simulink model "PROGRAM_COUNTER_02"  (R2022a)
settings: Solver=VariableStepAuto  StartTime=0.0  StopTime=10.0  RelTol=1e-3
undefined symbols (not defined in the file or in its folder): xc7z010iclg225
libraries: hdlBasic x1933, hlsBasic x1, vmcUtilities x1
(part 9 of 12)

== system PROGRAM_COUNTER_02/SUMADOR_64_BITS_1/ALU_SUM_18 ==
  CARRY_IN (1 BIT) : Inport
  A_INPUT (1 BIT) : Inport  Port=2
  B_INPUT (1 BIT) : Inport  Port=3
  Inverter1 : hdlBasic/Inverter  en=off  latency=0  XmcBlockStatus=1  maskContainerNames=group2  block_type=inv  block_config=sysgen:Inverter_config
  Inverter8 : hdlBasic/Inverter  en=off  latency=0  XmcBlockStatus=1  maskContainerNames=group2  block_type=inv  block_config=sysgen:Inverter_config
  Inverter9 : hdlBasic/Inverter  en=off  latency=0  XmcBlockStatus=1  maskContainerNames=group2  block_type=inv  block_config=sysgen:Inverter_config
  Logical : hdlBasic/Logical  logical_function=AND  inputs=2  en=off  latency=0  precision=Full  arith_type=Unsigned  n_bits=16  bin_pt=0  align_bp=on  overflow=[]  quantization=[]  XmcBlockStatus=1  maskContainerNames=tabcontainer1  block_type=logical  block_config=sysgen:Logical_config
  Logical1 : hdlBasic/Logical  logical_function=AND  inputs=2  en=off  latency=0  precision=Full  arith_type=Unsigned  n_bits=16  bin_pt=0  align_bp=on  overflow=[]  quantization=[]  XmcBlockStatus=1  maskContainerNames=tabcontainer1  block_type=logical  block_config=sysgen:Logical_config
  Logical2 : hdlBasic/Logical  logical_function=AND  inputs=2  en=off  latency=0  precision=Full  arith_type=Unsigned  n_bits=16  bin_pt=0  align_bp=on  overflow=[]  quantization=[]  XmcBlockStatus=1  maskContainerNames=tabcontainer1  block_type=logical  block_config=sysgen:Logical_config
  Logical{4..6,9} (4 alike) : hdlBasic/Logical  logical_function=AND  inputs=3  en=off  latency=0  precision=Full  arith_type=Unsigned  n_bits=16  bin_pt=0  align_bp=on  overflow=[]  quantization=[]  XmcBlockStatus=1  maskContainerNames=tabcontainer1  block_type=logical  block_config=sysgen:Logical_config
  Sum : hdlBasic/Logical  logical_function=OR  inputs=4  en=off  latency=0  precision=Full  arith_type=Unsigned  n_bits=16  bin_pt=0  align_bp=on  overflow=[]  quantization=[]  XmcBlockStatus=1  maskContainerNames=tabcontainer1  block_type=logical  block_config=sysgen:Logical_config
  c_out : hdlBasic/Logical  logical_function=OR  inputs=3  en=off  latency=0  precision=Full  arith_type=Unsigned  n_bits=16  bin_pt=0  align_bp=on  overflow=[]  quantization=[]  XmcBlockStatus=1  maskContainerNames=tabcontainer1  block_type=logical  block_config=sysgen:Logical_config
  ALU_OUT (1 BIT) : Outport
  CARRY_OUT (1 BIT) : Outport  Port=2
  wires:
  A_INPUT (1 BIT)/1 -> Inverter8/1, Logical5/2, Logical/2, Logical2/1, Logical9/2
  Logical1/1 -> c_out/2
  Inverter8/1 -> Logical6/2, Logical4/2
  CARRY_IN (1 BIT)/1 -> Inverter1/1, Logical5/1, Logical4/1, Logical1/1, Logical/1
  B_INPUT (1 BIT)/1 -> Logical5/3, Logical6/3, Logical1/2, Logical2/2, Inverter9/1
  Inverter1/1 -> Logical6/1, Logical9/1
  Logical6/1 -> Sum/3
  Logical9/1 -> Sum/2
  Logical4/1 -> Sum/1
  Logical/1 -> c_out/1
  Logical5/1 -> Sum/4
  Inverter9/1 -> Logical9/3, Logical4/3
  Sum/1 -> ALU_OUT (1 BIT)/1
  Logical2/1 -> c_out/3
  c_out/1 -> CARRY_OUT (1 BIT)/1

== system PROGRAM_COUNTER_02/SUMADOR_64_BITS_1/ALU_SUM_19 ==
  CARRY_IN (1 BIT) : Inport
  A_INPUT (1 BIT) : Inport  Port=2
  B_INPUT (1 BIT) : Inport  Port=3
  Inverter1 : hdlBasic/Inverter  en=off  latency=0  XmcBlockStatus=1  maskContainerNames=group2  block_type=inv  block_config=sysgen:Inverter_config
  Inverter8 : hdlBasic/Inverter  en=off  latency=0  XmcBlockStatus=1  maskContainerNames=group2  block_type=inv  block_config=sysgen:Inverter_config
  Inverter9 : hdlBasic/Inverter  en=off  latency=0  XmcBlockStatus=1  maskContainerNames=group2  block_type=inv  block_config=sysgen:Inverter_config
  Logical : hdlBasic/Logical  logical_function=AND  inputs=2  en=off  latency=0  precision=Full  arith_type=Unsigned  n_bits=16  bin_pt=0  align_bp=on  overflow=[]  quantization=[]  XmcBlockStatus=1  maskContainerNames=tabcontainer1  block_type=logical  block_config=sysgen:Logical_config
  Logical1 : hdlBasic/Logical  logical_function=AND  inputs=2  en=off  latency=0  precision=Full  arith_type=Unsigned  n_bits=16  bin_pt=0  align_bp=on  overflow=[]  quantization=[]  XmcBlockStatus=1  maskContainerNames=tabcontainer1  block_type=logical  block_config=sysgen:Logical_config
  Logical2 : hdlBasic/Logical  logical_function=AND  inputs=2  en=off  latency=0  precision=Full  arith_type=Unsigned  n_bits=16  bin_pt=0  align_bp=on  overflow=[]  quantization=[]  XmcBlockStatus=1  maskContainerNames=tabcontainer1  block_type=logical  block_config=sysgen:Logical_config
  Logical{4..6,9} (4 alike) : hdlBasic/Logical  logical_function=AND  inputs=3  en=off  latency=0  precision=Full  arith_type=Unsigned  n_bits=16  bin_pt=0  align_bp=on  overflow=[]  quantization=[]  XmcBlockStatus=1  maskContainerNames=tabcontainer1  block_type=logical  block_config=sysgen:Logical_config
  Sum : hdlBasic/Logical  logical_function=OR  inputs=4  en=off  latency=0  precision=Full  arith_type=Unsigned  n_bits=16  bin_pt=0  align_bp=on  overflow=[]  quantization=[]  XmcBlockStatus=1  maskContainerNames=tabcontainer1  block_type=logical  block_config=sysgen:Logical_config
  c_out : hdlBasic/Logical  logical_function=OR  inputs=3  en=off  latency=0  precision=Full  arith_type=Unsigned  n_bits=16  bin_pt=0  align_bp=on  overflow=[]  quantization=[]  XmcBlockStatus=1  maskContainerNames=tabcontainer1  block_type=logical  block_config=sysgen:Logical_config
  ALU_OUT (1 BIT) : Outport
  CARRY_OUT (1 BIT) : Outport  Port=2
  wires:
  A_INPUT (1 BIT)/1 -> Inverter8/1, Logical5/2, Logical/2, Logical2/1, Logical9/2
  Logical1/1 -> c_out/2
  Inverter8/1 -> Logical6/2, Logical4/2
  CARRY_IN (1 BIT)/1 -> Inverter1/1, Logical5/1, Logical4/1, Logical1/1, Logical/1
  B_INPUT (1 BIT)/1 -> Logical5/3, Logical6/3, Logical1/2, Logical2/2, Inverter9/1
  Inverter1/1 -> Logical6/1, Logical9/1
  Logical6/1 -> Sum/3
  Logical9/1 -> Sum/2
  Logical4/1 -> Sum/1
  Logical/1 -> c_out/1
  Logical5/1 -> Sum/4
  Inverter9/1 -> Logical9/3, Logical4/3
  Sum/1 -> ALU_OUT (1 BIT)/1
  Logical2/1 -> c_out/3
  c_out/1 -> CARRY_OUT (1 BIT)/1

== system PROGRAM_COUNTER_02/SUMADOR_64_BITS_1/ALU_SUM_2 ==
  CARRY_IN (1 BIT) : Inport
  A_INPUT (1 BIT) : Inport  Port=2
  B_INPUT (1 BIT) : Inport  Port=3
  Inverter1 : hdlBasic/Inverter  en=off  latency=0  XmcBlockStatus=1  maskContainerNames=group2  block_type=inv  block_config=sysgen:Inverter_config
  Inverter8 : hdlBasic/Inverter  en=off  latency=0  XmcBlockStatus=1  maskContainerNames=group2  block_type=inv  block_config=sysgen:Inverter_config
  Inverter9 : hdlBasic/Inverter  en=off  latency=0  XmcBlockStatus=1  maskContainerNames=group2  block_type=inv  block_config=sysgen:Inverter_config
  Logical : hdlBasic/Logical  logical_function=AND  inputs=2  en=off  latency=0  precision=Full  arith_type=Unsigned  n_bits=16  bin_pt=0  align_bp=on  overflow=[]  quantization=[]  XmcBlockStatus=1  maskContainerNames=tabcontainer1  block_type=logical  block_config=sysgen:Logical_config
  Logical1 : hdlBasic/Logical  logical_function=AND  inputs=2  en=off  latency=0  precision=Full  arith_type=Unsigned  n_bits=16  bin_pt=0  align_bp=on  overflow=[]  quantization=[]  XmcBlockStatus=1  maskContainerNames=tabcontainer1  block_type=logical  block_config=sysgen:Logical_config
  Logical2 : hdlBasic/Logical  logical_function=AND  inputs=2  en=off  latency=0  precision=Full  arith_type=Unsigned  n_bits=16  bin_pt=0  align_bp=on  overflow=[]  quantization=[]  XmcBlockStatus=1  maskContainerNames=tabcontainer1  block_type=logical  block_config=sysgen:Logical_config
  Logical{4..6,9} (4 alike) : hdlBasic/Logical  logical_function=AND  inputs=3  en=off  latency=0  precision=Full  arith_type=Unsigned  n_bits=16  bin_pt=0  align_bp=on  overflow=[]  quantization=[]  XmcBlockStatus=1  maskContainerNames=tabcontainer1  block_type=logical  block_config=sysgen:Logical_config
  Sum : hdlBasic/Logical  logical_function=OR  inputs=4  en=off  latency=0  precision=Full  arith_type=Unsigned  n_bits=16  bin_pt=0  align_bp=on  overflow=[]  quantization=[]  XmcBlockStatus=1  maskContainerNames=tabcontainer1  block_type=logical  block_config=sysgen:Logical_config
  c_out : hdlBasic/Logical  logical_function=OR  inputs=3  en=off  latency=0  precision=Full  arith_type=Unsigned  n_bits=16  bin_pt=0  align_bp=on  overflow=[]  quantization=[]  XmcBlockStatus=1  maskContainerNames=tabcontainer1  block_type=logical  block_config=sysgen:Logical_config
  ALU_OUT (1 BIT) : Outport
  CARRY_OUT (1 BIT) : Outport  Port=2
  wires:
  A_INPUT (1 BIT)/1 -> Inverter8/1, Logical5/2, Logical/2, Logical2/1, Logical9/2
  Logical1/1 -> c_out/2
  Inverter8/1 -> Logical6/2, Logical4/2
  CARRY_IN (1 BIT)/1 -> Inverter1/1, Logical5/1, Logical4/1, Logical1/1, Logical/1
  B_INPUT (1 BIT)/1 -> Logical5/3, Logical6/3, Logical1/2, Logical2/2, Inverter9/1
  Inverter1/1 -> Logical6/1, Logical9/1
  Logical6/1 -> Sum/3
  Logical9/1 -> Sum/2
  Logical4/1 -> Sum/1
  Logical/1 -> c_out/1
  Logical5/1 -> Sum/4
  Inverter9/1 -> Logical9/3, Logical4/3
  Sum/1 -> ALU_OUT (1 BIT)/1
  Logical2/1 -> c_out/3
  c_out/1 -> CARRY_OUT (1 BIT)/1

== system PROGRAM_COUNTER_02/SUMADOR_64_BITS_1/ALU_SUM_20 ==
  CARRY_IN (1 BIT) : Inport
  A_INPUT (1 BIT) : Inport  Port=2
  B_INPUT (1 BIT) : Inport  Port=3
  Inverter1 : hdlBasic/Inverter  en=off  latency=0  XmcBlockStatus=1  maskContainerNames=group2  block_type=inv  block_config=sysgen:Inverter_config
  Inverter8 : hdlBasic/Inverter  en=off  latency=0  XmcBlockStatus=1  maskContainerNames=group2  block_type=inv  block_config=sysgen:Inverter_config
  Inverter9 : hdlBasic/Inverter  en=off  latency=0  XmcBlockStatus=1  maskContainerNames=group2  block_type=inv  block_config=sysgen:Inverter_config
  Logical : hdlBasic/Logical  logical_function=AND  inputs=2  en=off  latency=0  precision=Full  arith_type=Unsigned  n_bits=16  bin_pt=0  align_bp=on  overflow=[]  quantization=[]  XmcBlockStatus=1  maskContainerNames=tabcontainer1  block_type=logical  block_config=sysgen:Logical_config
  Logical1 : hdlBasic/Logical  logical_function=AND  inputs=2  en=off  latency=0  precision=Full  arith_type=Unsigned  n_bits=16  bin_pt=0  align_bp=on  overflow=[]  quantization=[]  XmcBlockStatus=1  maskContainerNames=tabcontainer1  block_type=logical  block_config=sysgen:Logical_config
  Logical2 : hdlBasic/Logical  logical_function=AND  inputs=2  en=off  latency=0  precision=Full  arith_type=Unsigned  n_bits=16  bin_pt=0  align_bp=on  overflow=[]  quantization=[]  XmcBlockStatus=1  maskContainerNames=tabcontainer1  block_type=logical  block_config=sysgen:Logical_config
  Logical{4..6,9} (4 alike) : hdlBasic/Logical  logical_function=AND  inputs=3  en=off  latency=0  precision=Full  arith_type=Unsigned  n_bits=16  bin_pt=0  align_bp=on  overflow=[]  quantization=[]  XmcBlockStatus=1  maskContainerNames=tabcontainer1  block_type=logical  block_config=sysgen:Logical_config
  Sum : hdlBasic/Logical  logical_function=OR  inputs=4  en=off  latency=0  precision=Full  arith_type=Unsigned  n_bits=16  bin_pt=0  align_bp=on  overflow=[]  quantization=[]  XmcBlockStatus=1  maskContainerNames=tabcontainer1  block_type=logical  block_config=sysgen:Logical_config
  c_out : hdlBasic/Logical  logical_function=OR  inputs=3  en=off  latency=0  precision=Full  arith_type=Unsigned  n_bits=16  bin_pt=0  align_bp=on  overflow=[]  quantization=[]  XmcBlockStatus=1  maskContainerNames=tabcontainer1  block_type=logical  block_config=sysgen:Logical_config
  ALU_OUT (1 BIT) : Outport
  CARRY_OUT (1 BIT) : Outport  Port=2
  wires:
  A_INPUT (1 BIT)/1 -> Inverter8/1, Logical5/2, Logical/2, Logical2/1, Logical9/2
  Logical1/1 -> c_out/2
  Inverter8/1 -> Logical6/2, Logical4/2
  CARRY_IN (1 BIT)/1 -> Inverter1/1, Logical5/1, Logical4/1, Logical1/1, Logical/1
  B_INPUT (1 BIT)/1 -> Logical5/3, Logical6/3, Logical1/2, Logical2/2, Inverter9/1
  Inverter1/1 -> Logical6/1, Logical9/1
  Logical6/1 -> Sum/3
  Logical9/1 -> Sum/2
  Logical4/1 -> Sum/1
  Logical/1 -> c_out/1
  Logical5/1 -> Sum/4
  Inverter9/1 -> Logical9/3, Logical4/3
  Sum/1 -> ALU_OUT (1 BIT)/1
  Logical2/1 -> c_out/3
  c_out/1 -> CARRY_OUT (1 BIT)/1

== system PROGRAM_COUNTER_02/SUMADOR_64_BITS_1/ALU_SUM_21 ==
  CARRY_IN (1 BIT) : Inport
  A_INPUT (1 BIT) : Inport  Port=2
  B_INPUT (1 BIT) : Inport  Port=3
  Inverter1 : hdlBasic/Inverter  en=off  latency=0  XmcBlockStatus=1  maskContainerNames=group2  block_type=inv  block_config=sysgen:Inverter_config
  Inverter8 : hdlBasic/Inverter  en=off  latency=0  XmcBlockStatus=1  maskContainerNames=group2  block_type=inv  block_config=sysgen:Inverter_config
  Inverter9 : hdlBasic/Inverter  en=off  latency=0  XmcBlockStatus=1  maskContainerNames=group2  block_type=inv  block_config=sysgen:Inverter_config
  Logical : hdlBasic/Logical  logical_function=AND  inputs=2  en=off  latency=0  precision=Full  arith_type=Unsigned  n_bits=16  bin_pt=0  align_bp=on  overflow=[]  quantization=[]  XmcBlockStatus=1  maskContainerNames=tabcontainer1  block_type=logical  block_config=sysgen:Logical_config
  Logical1 : hdlBasic/Logical  logical_function=AND  inputs=2  en=off  latency=0  precision=Full  arith_type=Unsigned  n_bits=16  bin_pt=0  align_bp=on  overflow=[]  quantization=[]  XmcBlockStatus=1  maskContainerNames=tabcontainer1  block_type=logical  block_config=sysgen:Logical_config
  Logical2 : hdlBasic/Logical  logical_function=AND  inputs=2  en=off  latency=0  precision=Full  arith_type=Unsigned  n_bits=16  bin_pt=0  align_bp=on  overflow=[]  quantization=[]  XmcBlockStatus=1  maskContainerNames=tabcontainer1  block_type=logical  block_config=sysgen:Logical_config
  Logical{4..6,9} (4 alike) : hdlBasic/Logical  logical_function=AND  inputs=3  en=off  latency=0  precision=Full  arith_type=Unsigned  n_bits=16  bin_pt=0  align_bp=on  overflow=[]  quantization=[]  XmcBlockStatus=1  maskContainerNames=tabcontainer1  block_type=logical  block_config=sysgen:Logical_config
  Sum : hdlBasic/Logical  logical_function=OR  inputs=4  en=off  latency=0  precision=Full  arith_type=Unsigned  n_bits=16  bin_pt=0  align_bp=on  overflow=[]  quantization=[]  XmcBlockStatus=1  maskContainerNames=tabcontainer1  block_type=logical  block_config=sysgen:Logical_config
  c_out : hdlBasic/Logical  logical_function=OR  inputs=3  en=off  latency=0  precision=Full  arith_type=Unsigned  n_bits=16  bin_pt=0  align_bp=on  overflow=[]  quantization=[]  XmcBlockStatus=1  maskContainerNames=tabcontainer1  block_type=logical  block_config=sysgen:Logical_config
  ALU_OUT (1 BIT) : Outport
  CARRY_OUT (1 BIT) : Outport  Port=2
  wires:
  A_INPUT (1 BIT)/1 -> Inverter8/1, Logical5/2, Logical/2, Logical2/1, Logical9/2
  Logical1/1 -> c_out/2
  Inverter8/1 -> Logical6/2, Logical4/2
  CARRY_IN (1 BIT)/1 -> Inverter1/1, Logical5/1, Logical4/1, Logical1/1, Logical/1
  B_INPUT (1 BIT)/1 -> Logical5/3, Logical6/3, Logical1/2, Logical2/2, Inverter9/1
  Inverter1/1 -> Logical6/1, Logical9/1
  Logical6/1 -> Sum/3
  Logical9/1 -> Sum/2
  Logical4/1 -> Sum/1
  Logical/1 -> c_out/1
  Logical5/1 -> Sum/4
  Inverter9/1 -> Logical9/3, Logical4/3
  Sum/1 -> ALU_OUT (1 BIT)/1
  Logical2/1 -> c_out/3
  c_out/1 -> CARRY_OUT (1 BIT)/1

== system PROGRAM_COUNTER_02/SUMADOR_64_BITS_1/ALU_SUM_22 ==
  CARRY_IN (1 BIT) : Inport
  A_INPUT (1 BIT) : Inport  Port=2
  B_INPUT (1 BIT) : Inport  Port=3
  Inverter1 : hdlBasic/Inverter  en=off  latency=0  XmcBlockStatus=1  maskContainerNames=group2  block_type=inv  block_config=sysgen:Inverter_config
  Inverter8 : hdlBasic/Inverter  en=off  latency=0  XmcBlockStatus=1  maskContainerNames=group2  block_type=inv  block_config=sysgen:Inverter_config
  Inverter9 : hdlBasic/Inverter  en=off  latency=0  XmcBlockStatus=1  maskContainerNames=group2  block_type=inv  block_config=sysgen:Inverter_config
  Logical : hdlBasic/Logical  logical_function=AND  inputs=2  en=off  latency=0  precision=Full  arith_type=Unsigned  n_bits=16  bin_pt=0  align_bp=on  overflow=[]  quantization=[]  XmcBlockStatus=1  maskContainerNames=tabcontainer1  block_type=logical  block_config=sysgen:Logical_config
  Logical1 : hdlBasic/Logical  logical_function=AND  inputs=2  en=off  latency=0  precision=Full  arith_type=Unsigned  n_bits=16  bin_pt=0  align_bp=on  overflow=[]  quantization=[]  XmcBlockStatus=1  maskContainerNames=tabcontainer1  block_type=logical  block_config=sysgen:Logical_config
  Logical2 : hdlBasic/Logical  logical_function=AND  inputs=2  en=off  latency=0  precision=Full  arith_type=Unsigned  n_bits=16  bin_pt=0  align_bp=on  overflow=[]  quantization=[]  XmcBlockStatus=1  maskContainerNames=tabcontainer1  block_type=logical  block_config=sysgen:Logical_config
  Logical{4..6,9} (4 alike) : hdlBasic/Logical  logical_function=AND  inputs=3  en=off  latency=0  precision=Full  arith_type=Unsigned  n_bits=16  bin_pt=0  align_bp=on  overflow=[]  quantization=[]  XmcBlockStatus=1  maskContainerNames=tabcontainer1  block_type=logical  block_config=sysgen:Logical_config
  Sum : hdlBasic/Logical  logical_function=OR  inputs=4  en=off  latency=0  precision=Full  arith_type=Unsigned  n_bits=16  bin_pt=0  align_bp=on  overflow=[]  quantization=[]  XmcBlockStatus=1  maskContainerNames=tabcontainer1  block_type=logical  block_config=sysgen:Logical_config
  c_out : hdlBasic/Logical  logical_function=OR  inputs=3  en=off  latency=0  precision=Full  arith_type=Unsigned  n_bits=16  bin_pt=0  align_bp=on  overflow=[]  quantization=[]  XmcBlockStatus=1  maskContainerNames=tabcontainer1  block_type=logical  block_config=sysgen:Logical_config
  ALU_OUT (1 BIT) : Outport
  CARRY_OUT (1 BIT) : Outport  Port=2
  wires:
  A_INPUT (1 BIT)/1 -> Inverter8/1, Logical5/2, Logical/2, Logical2/1, Logical9/2
  Logical1/1 -> c_out/2
  Inverter8/1 -> Logical6/2, Logical4/2
  CARRY_IN (1 BIT)/1 -> Inverter1/1, Logical5/1, Logical4/1, Logical1/1, Logical/1
  B_INPUT (1 BIT)/1 -> Logical5/3, Logical6/3, Logical1/2, Logical2/2, Inverter9/1
  Inverter1/1 -> Logical6/1, Logical9/1
  Logical6/1 -> Sum/3
  Logical9/1 -> Sum/2
  Logical4/1 -> Sum/1
  Logical/1 -> c_out/1
  Logical5/1 -> Sum/4
  Inverter9/1 -> Logical9/3, Logical4/3
  Sum/1 -> ALU_OUT (1 BIT)/1
  Logical2/1 -> c_out/3
  c_out/1 -> CARRY_OUT (1 BIT)/1

== system PROGRAM_COUNTER_02/SUMADOR_64_BITS_1/ALU_SUM_23 ==
  CARRY_IN (1 BIT) : Inport
  A_INPUT (1 BIT) : Inport  Port=2
  B_INPUT (1 BIT) : Inport  Port=3
  Inverter1 : hdlBasic/Inverter  en=off  latency=0  XmcBlockStatus=1  maskContainerNames=group2  block_type=inv  block_config=sysgen:Inverter_config
  Inverter8 : hdlBasic/Inverter  en=off  latency=0  XmcBlockStatus=1  maskContainerNames=group2  block_type=inv  block_config=sysgen:Inverter_config
  Inverter9 : hdlBasic/Inverter  en=off  latency=0  XmcBlockStatus=1  maskContainerNames=group2  block_type=inv  block_config=sysgen:Inverter_config
  Logical : hdlBasic/Logical  logical_function=AND  inputs=2  en=off  latency=0  precision=Full  arith_type=Unsigned  n_bits=16  bin_pt=0  align_bp=on  overflow=[]  quantization=[]  XmcBlockStatus=1  maskContainerNames=tabcontainer1  block_type=logical  block_config=sysgen:Logical_config
  Logical1 : hdlBasic/Logical  logical_function=AND  inputs=2  en=off  latency=0  precision=Full  arith_type=Unsigned  n_bits=16  bin_pt=0  align_bp=on  overflow=[]  quantization=[]  XmcBlockStatus=1  maskContainerNames=tabcontainer1  block_type=logical  block_config=sysgen:Logical_config
  Logical2 : hdlBasic/Logical  logical_function=AND  inputs=2  en=off  latency=0  precision=Full  arith_type=Unsigned  n_bits=16  bin_pt=0  align_bp=on  overflow=[]  quantization=[]  XmcBlockStatus=1  maskContainerNames=tabcontainer1  block_type=logical  block_config=sysgen:Logical_config
  Logical{4..6,9} (4 alike) : hdlBasic/Logical  logical_function=AND  inputs=3  en=off  latency=0  precision=Full  arith_type=Unsigned  n_bits=16  bin_pt=0  align_bp=on  overflow=[]  quantization=[]  XmcBlockStatus=1  maskContainerNames=tabcontainer1  block_type=logical  block_config=sysgen:Logical_config
  Sum : hdlBasic/Logical  logical_function=OR  inputs=4  en=off  latency=0  precision=Full  arith_type=Unsigned  n_bits=16  bin_pt=0  align_bp=on  overflow=[]  quantization=[]  XmcBlockStatus=1  maskContainerNames=tabcontainer1  block_type=logical  block_config=sysgen:Logical_config
  c_out : hdlBasic/Logical  logical_function=OR  inputs=3  en=off  latency=0  precision=Full  arith_type=Unsigned  n_bits=16  bin_pt=0  align_bp=on  overflow=[]  quantization=[]  XmcBlockStatus=1  maskContainerNames=tabcontainer1  block_type=logical  block_config=sysgen:Logical_config
  ALU_OUT (1 BIT) : Outport
  CARRY_OUT (1 BIT) : Outport  Port=2
  wires:
  A_INPUT (1 BIT)/1 -> Inverter8/1, Logical5/2, Logical/2, Logical2/1, Logical9/2
  Logical1/1 -> c_out/2
  Inverter8/1 -> Logical6/2, Logical4/2
  CARRY_IN (1 BIT)/1 -> Inverter1/1, Logical5/1, Logical4/1, Logical1/1, Logical/1
  B_INPUT (1 BIT)/1 -> Logical5/3, Logical6/3, Logical1/2, Logical2/2, Inverter9/1
  Inverter1/1 -> Logical6/1, Logical9/1
  Logical6/1 -> Sum/3
  Logical9/1 -> Sum/2
  Logical4/1 -> Sum/1
  Logical/1 -> c_out/1
  Logical5/1 -> Sum/4
  Inverter9/1 -> Logical9/3, Logical4/3
  Sum/1 -> ALU_OUT (1 BIT)/1
  Logical2/1 -> c_out/3
  c_out/1 -> CARRY_OUT (1 BIT)/1

== system PROGRAM_COUNTER_02/SUMADOR_64_BITS_1/ALU_SUM_24 ==
  CARRY_IN (1 BIT) : Inport
  A_INPUT (1 BIT) : Inport  Port=2
  B_INPUT (1 BIT) : Inport  Port=3
  Inverter1 : hdlBasic/Inverter  en=off  latency=0  XmcBlockStatus=1  maskContainerNames=group2  block_type=inv  block_config=sysgen:Inverter_config
  Inverter8 : hdlBasic/Inverter  en=off  latency=0  XmcBlockStatus=1  maskContainerNames=group2  block_type=inv  block_config=sysgen:Inverter_config
  Inverter9 : hdlBasic/Inverter  en=off  latency=0  XmcBlockStatus=1  maskContainerNames=group2  block_type=inv  block_config=sysgen:Inverter_config
  Logical : hdlBasic/Logical  logical_function=AND  inputs=2  en=off  latency=0  precision=Full  arith_type=Unsigned  n_bits=16  bin_pt=0  align_bp=on  overflow=[]  quantization=[]  XmcBlockStatus=1  maskContainerNames=tabcontainer1  block_type=logical  block_config=sysgen:Logical_config
  Logical1 : hdlBasic/Logical  logical_function=AND  inputs=2  en=off  latency=0  precision=Full  arith_type=Unsigned  n_bits=16  bin_pt=0  align_bp=on  overflow=[]  quantization=[]  XmcBlockStatus=1  maskContainerNames=tabcontainer1  block_type=logical  block_config=sysgen:Logical_config
  Logical2 : hdlBasic/Logical  logical_function=AND  inputs=2  en=off  latency=0  precision=Full  arith_type=Unsigned  n_bits=16  bin_pt=0  align_bp=on  overflow=[]  quantization=[]  XmcBlockStatus=1  maskContainerNames=tabcontainer1  block_type=logical  block_config=sysgen:Logical_config
  Logical{4..6,9} (4 alike) : hdlBasic/Logical  logical_function=AND  inputs=3  en=off  latency=0  precision=Full  arith_type=Unsigned  n_bits=16  bin_pt=0  align_bp=on  overflow=[]  quantization=[]  XmcBlockStatus=1  maskContainerNames=tabcontainer1  block_type=logical  block_config=sysgen:Logical_config
  Sum : hdlBasic/Logical  logical_function=OR  inputs=4  en=off  latency=0  precision=Full  arith_type=Unsigned  n_bits=16  bin_pt=0  align_bp=on  overflow=[]  quantization=[]  XmcBlockStatus=1  maskContainerNames=tabcontainer1  block_type=logical  block_config=sysgen:Logical_config
  c_out : hdlBasic/Logical  logical_function=OR  inputs=3  en=off  latency=0  precision=Full  arith_type=Unsigned  n_bits=16  bin_pt=0  align_bp=on  overflow=[]  quantization=[]  XmcBlockStatus=1  maskContainerNames=tabcontainer1  block_type=logical  block_config=sysgen:Logical_config
  ALU_OUT (1 BIT) : Outport
  CARRY_OUT (1 BIT) : Outport  Port=2
  wires:
  A_INPUT (1 BIT)/1 -> Inverter8/1, Logical5/2, Logical/2, Logical2/1, Logical9/2
  Logical1/1 -> c_out/2
  Inverter8/1 -> Logical6/2, Logical4/2
  CARRY_IN (1 BIT)/1 -> Inverter1/1, Logical5/1, Logical4/1, Logical1/1, Logical/1
  B_INPUT (1 BIT)/1 -> Logical5/3, Logical6/3, Logical1/2, Logical2/2, Inverter9/1
  Inverter1/1 -> Logical6/1, Logical9/1
  Logical6/1 -> Sum/3
  Logical9/1 -> Sum/2
  Logical4/1 -> Sum/1
  Logical/1 -> c_out/1
  Logical5/1 -> Sum/4
  Inverter9/1 -> Logical9/3, Logical4/3
  Sum/1 -> ALU_OUT (1 BIT)/1
  Logical2/1 -> c_out/3
  c_out/1 -> CARRY_OUT (1 BIT)/1

== system PROGRAM_COUNTER_02/SUMADOR_64_BITS_1/ALU_SUM_25 ==
  CARRY_IN (1 BIT) : Inport
  A_INPUT (1 BIT) : Inport  Port=2
  B_INPUT (1 BIT) : Inport  Port=3
  Inverter1 : hdlBasic/Inverter  en=off  latency=0  XmcBlockStatus=1  maskContainerNames=group2  block_type=inv  block_config=sysgen:Inverter_config
  Inverter8 : hdlBasic/Inverter  en=off  latency=0  XmcBlockStatus=1  maskContainerNames=group2  block_type=inv  block_config=sysgen:Inverter_config
  Inverter9 : hdlBasic/Inverter  en=off  latency=0  XmcBlockStatus=1  maskContainerNames=group2  block_type=inv  block_config=sysgen:Inverter_config
  Logical : hdlBasic/Logical  logical_function=AND  inputs=2  en=off  latency=0  precision=Full  arith_type=Unsigned  n_bits=16  bin_pt=0  align_bp=on  overflow=[]  quantization=[]  XmcBlockStatus=1  maskContainerNames=tabcontainer1  block_type=logical  block_config=sysgen:Logical_config
  Logical1 : hdlBasic/Logical  logical_function=AND  inputs=2  en=off  latency=0  precision=Full  arith_type=Unsigned  n_bits=16  bin_pt=0  align_bp=on  overflow=[]  quantization=[]  XmcBlockStatus=1  maskContainerNames=tabcontainer1  block_type=logical  block_config=sysgen:Logical_config
  Logical2 : hdlBasic/Logical  logical_function=AND  inputs=2  en=off  latency=0  precision=Full  arith_type=Unsigned  n_bits=16  bin_pt=0  align_bp=on  overflow=[]  quantization=[]  XmcBlockStatus=1  maskContainerNames=tabcontainer1  block_type=logical  block_config=sysgen:Logical_config
  Logical{4..6,9} (4 alike) : hdlBasic/Logical  logical_function=AND  inputs=3  en=off  latency=0  precision=Full  arith_type=Unsigned  n_bits=16  bin_pt=0  align_bp=on  overflow=[]  quantization=[]  XmcBlockStatus=1  maskContainerNames=tabcontainer1  block_type=logical  block_config=sysgen:Logical_config
  Sum : hdlBasic/Logical  logical_function=OR  inputs=4  en=off  latency=0  precision=Full  arith_type=Unsigned  n_bits=16  bin_pt=0  align_bp=on  overflow=[]  quantization=[]  XmcBlockStatus=1  maskContainerNames=tabcontainer1  block_type=logical  block_config=sysgen:Logical_config
  c_out : hdlBasic/Logical  logical_function=OR  inputs=3  en=off  latency=0  precision=Full  arith_type=Unsigned  n_bits=16  bin_pt=0  align_bp=on  overflow=[]  quantization=[]  XmcBlockStatus=1  maskContainerNames=tabcontainer1  block_type=logical  block_config=sysgen:Logical_config
  ALU_OUT (1 BIT) : Outport
  CARRY_OUT (1 BIT) : Outport  Port=2
  wires:
  A_INPUT (1 BIT)/1 -> Inverter8/1, Logical5/2, Logical/2, Logical2/1, Logical9/2
  Logical1/1 -> c_out/2
  Inverter8/1 -> Logical6/2, Logical4/2
  CARRY_IN (1 BIT)/1 -> Inverter1/1, Logical5/1, Logical4/1, Logical1/1, Logical/1
  B_INPUT (1 BIT)/1 -> Logical5/3, Logical6/3, Logical1/2, Logical2/2, Inverter9/1
  Inverter1/1 -> Logical6/1, Logical9/1
  Logical6/1 -> Sum/3
  Logical9/1 -> Sum/2
  Logical4/1 -> Sum/1
  Logical/1 -> c_out/1
  Logical5/1 -> Sum/4
  Inverter9/1 -> Logical9/3, Logical4/3
  Sum/1 -> ALU_OUT (1 BIT)/1
  Logical2/1 -> c_out/3
  c_out/1 -> CARRY_OUT (1 BIT)/1

== system PROGRAM_COUNTER_02/SUMADOR_64_BITS_1/ALU_SUM_26 ==
  CARRY_IN (1 BIT) : Inport
  A_INPUT (1 BIT) : Inport  Port=2
  B_INPUT (1 BIT) : Inport  Port=3
  Inverter1 : hdlBasic/Inverter  en=off  latency=0  XmcBlockStatus=1  maskContainerNames=group2  block_type=inv  block_config=sysgen:Inverter_config
  Inverter8 : hdlBasic/Inverter  en=off  latency=0  XmcBlockStatus=1  maskContainerNames=group2  block_type=inv  block_config=sysgen:Inverter_config
  Inverter9 : hdlBasic/Inverter  en=off  latency=0  XmcBlockStatus=1  maskContainerNames=group2  block_type=inv  block_config=sysgen:Inverter_config
  Logical : hdlBasic/Logical  logical_function=AND  inputs=2  en=off  latency=0  precision=Full  arith_type=Unsigned  n_bits=16  bin_pt=0  align_bp=on  overflow=[]  quantization=[]  XmcBlockStatus=1  maskContainerNames=tabcontainer1  block_type=logical  block_config=sysgen:Logical_config
  Logical1 : hdlBasic/Logical  logical_function=AND  inputs=2  en=off  latency=0  precision=Full  arith_type=Unsigned  n_bits=16  bin_pt=0  align_bp=on  overflow=[]  quantization=[]  XmcBlockStatus=1  maskContainerNames=tabcontainer1  block_type=logical  block_config=sysgen:Logical_config
  Logical2 : hdlBasic/Logical  logical_function=AND  inputs=2  en=off  latency=0  precision=Full  arith_type=Unsigned  n_bits=16  bin_pt=0  align_bp=on  overflow=[]  quantization=[]  XmcBlockStatus=1  maskContainerNames=tabcontainer1  block_type=logical  block_config=sysgen:Logical_config
  Logical{4..6,9} (4 alike) : hdlBasic/Logical  logical_function=AND  inputs=3  en=off  latency=0  precision=Full  arith_type=Unsigned  n_bits=16  bin_pt=0  align_bp=on  overflow=[]  quantization=[]  XmcBlockStatus=1  maskContainerNames=tabcontainer1  block_type=logical  block_config=sysgen:Logical_config
  Sum : hdlBasic/Logical  logical_function=OR  inputs=4  en=off  latency=0  precision=Full  arith_type=Unsigned  n_bits=16  bin_pt=0  align_bp=on  overflow=[]  quantization=[]  XmcBlockStatus=1  maskContainerNames=tabcontainer1  block_type=logical  block_config=sysgen:Logical_config
  c_out : hdlBasic/Logical  logical_function=OR  inputs=3  en=off  latency=0  precision=Full  arith_type=Unsigned  n_bits=16  bin_pt=0  align_bp=on  overflow=[]  quantization=[]  XmcBlockStatus=1  maskContainerNames=tabcontainer1  block_type=logical  block_config=sysgen:Logical_config
  ALU_OUT (1 BIT) : Outport
  CARRY_OUT (1 BIT) : Outport  Port=2
  wires:
  A_INPUT (1 BIT)/1 -> Inverter8/1, Logical5/2, Logical/2, Logical2/1, Logical9/2
  Logical1/1 -> c_out/2
  Inverter8/1 -> Logical6/2, Logical4/2
  CARRY_IN (1 BIT)/1 -> Inverter1/1, Logical5/1, Logical4/1, Logical1/1, Logical/1
  B_INPUT (1 BIT)/1 -> Logical5/3, Logical6/3, Logical1/2, Logical2/2, Inverter9/1
  Inverter1/1 -> Logical6/1, Logical9/1
  Logical6/1 -> Sum/3
  Logical9/1 -> Sum/2
  Logical4/1 -> Sum/1
  Logical/1 -> c_out/1
  Logical5/1 -> Sum/4
  Inverter9/1 -> Logical9/3, Logical4/3
  Sum/1 -> ALU_OUT (1 BIT)/1
  Logical2/1 -> c_out/3
  c_out/1 -> CARRY_OUT (1 BIT)/1

== system PROGRAM_COUNTER_02/SUMADOR_64_BITS_1/ALU_SUM_27 ==
  CARRY_IN (1 BIT) : Inport
  A_INPUT (1 BIT) : Inport  Port=2
  B_INPUT (1 BIT) : Inport  Port=3
  Inverter1 : hdlBasic/Inverter  en=off  latency=0  XmcBlockStatus=1  maskContainerNames=group2  block_type=inv  block_config=sysgen:Inverter_config
  Inverter8 : hdlBasic/Inverter  en=off  latency=0  XmcBlockStatus=1  maskContainerNames=group2  block_type=inv  block_config=sysgen:Inverter_config
  Inverter9 : hdlBasic/Inverter  en=off  latency=0  XmcBlockStatus=1  maskContainerNames=group2  block_type=inv  block_config=sysgen:Inverter_config
  Logical : hdlBasic/Logical  logical_function=AND  inputs=2  en=off  latency=0  precision=Full  arith_type=Unsigned  n_bits=16  bin_pt=0  align_bp=on  overflow=[]  quantization=[]  XmcBlockStatus=1  maskContainerNames=tabcontainer1  block_type=logical  block_config=sysgen:Logical_config
  Logical1 : hdlBasic/Logical  logical_function=AND  inputs=2  en=off  latency=0  precision=Full  arith_type=Unsigned  n_bits=16  bin_pt=0  align_bp=on  overflow=[]  quantization=[]  XmcBlockStatus=1  maskContainerNames=tabcontainer1  block_type=logical  block_config=sysgen:Logical_config
  Logical2 : hdlBasic/Logical  logical_function=AND  inputs=2  en=off  latency=0  precision=Full  arith_type=Unsigned  n_bits=16  bin_pt=0  align_bp=on  overflow=[]  quantization=[]  XmcBlockStatus=1  maskContainerNames=tabcontainer1  block_type=logical  block_config=sysgen:Logical_config
  Logical{4..6,9} (4 alike) : hdlBasic/Logical  logical_function=AND  inputs=3  en=off  latency=0  precision=Full  arith_type=Unsigned  n_bits=16  bin_pt=0  align_bp=on  overflow=[]  quantization=[]  XmcBlockStatus=1  maskContainerNames=tabcontainer1  block_type=logical  block_config=sysgen:Logical_config
  Sum : hdlBasic/Logical  logical_function=OR  inputs=4  en=off  latency=0  precision=Full  arith_type=Unsigned  n_bits=16  bin_pt=0  align_bp=on  overflow=[]  quantization=[]  XmcBlockStatus=1  maskContainerNames=tabcontainer1  block_type=logical  block_config=sysgen:Logical_config
  c_out : hdlBasic/Logical  logical_function=OR  inputs=3  en=off  latency=0  precision=Full  arith_type=Unsigned  n_bits=16  bin_pt=0  align_bp=on  overflow=[]  quantization=[]  XmcBlockStatus=1  maskContainerNames=tabcontainer1  block_type=logical  block_config=sysgen:Logical_config
  ALU_OUT (1 BIT) : Outport
  CARRY_OUT (1 BIT) : Outport  Port=2
  wires:
  A_INPUT (1 BIT)/1 -> Inverter8/1, Logical5/2, Logical/2, Logical2/1, Logical9/2
  Logical1/1 -> c_out/2
  Inverter8/1 -> Logical6/2, Logical4/2
  CARRY_IN (1 BIT)/1 -> Inverter1/1, Logical5/1, Logical4/1, Logical1/1, Logical/1
  B_INPUT (1 BIT)/1 -> Logical5/3, Logical6/3, Logical1/2, Logical2/2, Inverter9/1
  Inverter1/1 -> Logical6/1, Logical9/1
  Logical6/1 -> Sum/3
  Logical9/1 -> Sum/2
  Logical4/1 -> Sum/1
  Logical/1 -> c_out/1
  Logical5/1 -> Sum/4
  Inverter9/1 -> Logical9/3, Logical4/3
  Sum/1 -> ALU_OUT (1 BIT)/1
  Logical2/1 -> c_out/3
  c_out/1 -> CARRY_OUT (1 BIT)/1

== system PROGRAM_COUNTER_02/SUMADOR_64_BITS_1/ALU_SUM_28 ==
  CARRY_IN (1 BIT) : Inport
  A_INPUT (1 BIT) : Inport  Port=2
  B_INPUT (1 BIT) : Inport  Port=3
  Inverter1 : hdlBasic/Inverter  en=off  latency=0  XmcBlockStatus=1  maskContainerNames=group2  block_type=inv  block_config=sysgen:Inverter_config
  Inverter8 : hdlBasic/Inverter  en=off  latency=0  XmcBlockStatus=1  maskContainerNames=group2  block_type=inv  block_config=sysgen:Inverter_config
  Inverter9 : hdlBasic/Inverter  en=off  latency=0  XmcBlockStatus=1  maskContainerNames=group2  block_type=inv  block_config=sysgen:Inverter_config
  Logical : hdlBasic/Logical  logical_function=AND  inputs=2  en=off  latency=0  precision=Full  arith_type=Unsigned  n_bits=16  bin_pt=0  align_bp=on  overflow=[]  quantization=[]  XmcBlockStatus=1  maskContainerNames=tabcontainer1  block_type=logical  block_config=sysgen:Logical_config
  Logical1 : hdlBasic/Logical  logical_function=AND  inputs=2  en=off  latency=0  precision=Full  arith_type=Unsigned  n_bits=16  bin_pt=0  align_bp=on  overflow=[]  quantization=[]  XmcBlockStatus=1  maskContainerNames=tabcontainer1  block_type=logical  block_config=sysgen:Logical_config
  Logical2 : hdlBasic/Logical  logical_function=AND  inputs=2  en=off  latency=0  precision=Full  arith_type=Unsigned  n_bits=16  bin_pt=0  align_bp=on  overflow=[]  quantization=[]  XmcBlockStatus=1  maskContainerNames=tabcontainer1  block_type=logical  block_config=sysgen:Logical_config
  Logical{4..6,9} (4 alike) : hdlBasic/Logical  logical_function=AND  inputs=3  en=off  latency=0  precision=Full  arith_type=Unsigned  n_bits=16  bin_pt=0  align_bp=on  overflow=[]  quantization=[]  XmcBlockStatus=1  maskContainerNames=tabcontainer1  block_type=logical  block_config=sysgen:Logical_config
  Sum : hdlBasic/Logical  logical_function=OR  inputs=4  en=off  latency=0  precision=Full  arith_type=Unsigned  n_bits=16  bin_pt=0  align_bp=on  overflow=[]  quantization=[]  XmcBlockStatus=1  maskContainerNames=tabcontainer1  block_type=logical  block_config=sysgen:Logical_config
  c_out : hdlBasic/Logical  logical_function=OR  inputs=3  en=off  latency=0  precision=Full  arith_type=Unsigned  n_bits=16  bin_pt=0  align_bp=on  overflow=[]  quantization=[]  XmcBlockStatus=1  maskContainerNames=tabcontainer1  block_type=logical  block_config=sysgen:Logical_config
  ALU_OUT (1 BIT) : Outport
  CARRY_OUT (1 BIT) : Outport  Port=2
  wires:
  A_INPUT (1 BIT)/1 -> Inverter8/1, Logical5/2, Logical/2, Logical2/1, Logical9/2
  Logical1/1 -> c_out/2
  Inverter8/1 -> Logical6/2, Logical4/2
  CARRY_IN (1 BIT)/1 -> Inverter1/1, Logical5/1, Logical4/1, Logical1/1, Logical/1
  B_INPUT (1 BIT)/1 -> Logical5/3, Logical6/3, Logical1/2, Logical2/2, Inverter9/1
  Inverter1/1 -> Logical6/1, Logical9/1
  Logical6/1 -> Sum/3
  Logical9/1 -> Sum/2
  Logical4/1 -> Sum/1
  Logical/1 -> c_out/1
  Logical5/1 -> Sum/4
  Inverter9/1 -> Logical9/3, Logical4/3
  Sum/1 -> ALU_OUT (1 BIT)/1
  Logical2/1 -> c_out/3
  c_out/1 -> CARRY_OUT (1 BIT)/1

== system PROGRAM_COUNTER_02/SUMADOR_64_BITS_1/ALU_SUM_29 ==
  CARRY_IN (1 BIT) : Inport
  A_INPUT (1 BIT) : Inport  Port=2
  B_INPUT (1 BIT) : Inport  Port=3
  Inverter1 : hdlBasic/Inverter  en=off  latency=0  XmcBlockStatus=1  maskContainerNames=group2  block_type=inv  block_config=sysgen:Inverter_config
  Inverter8 : hdlBasic/Inverter  en=off  latency=0  XmcBlockStatus=1  maskContainerNames=group2  block_type=inv  block_config=sysgen:Inverter_config
  Inverter9 : hdlBasic/Inverter  en=off  latency=0  XmcBlockStatus=1  maskContainerNames=group2  block_type=inv  block_config=sysgen:Inverter_config
  Logical : hdlBasic/Logical  logical_function=AND  inputs=2  en=off  latency=0  precision=Full  arith_type=Unsigned  n_bits=16  bin_pt=0  align_bp=on  overflow=[]  quantization=[]  XmcBlockStatus=1  maskContainerNames=tabcontainer1  block_type=logical  block_config=sysgen:Logical_config
  Logical1 : hdlBasic/Logical  logical_function=AND  inputs=2  en=off  latency=0  precision=Full  arith_type=Unsigned  n_bits=16  bin_pt=0  align_bp=on  overflow=[]  quantization=[]  XmcBlockStatus=1  maskContainerNames=tabcontainer1  block_type=logical  block_config=sysgen:Logical_config
  Logical2 : hdlBasic/Logical  logical_function=AND  inputs=2  en=off  latency=0  precision=Full  arith_type=Unsigned  n_bits=16  bin_pt=0  align_bp=on  overflow=[]  quantization=[]  XmcBlockStatus=1  maskContainerNames=tabcontainer1  block_type=logical  block_config=sysgen:Logical_config
  Logical{4..6,9} (4 alike) : hdlBasic/Logical  logical_function=AND  inputs=3  en=off  latency=0  precision=Full  arith_type=Unsigned  n_bits=16  bin_pt=0  align_bp=on  overflow=[]  quantization=[]  XmcBlockStatus=1  maskContainerNames=tabcontainer1  block_type=logical  block_config=sysgen:Logical_config
  Sum : hdlBasic/Logical  logical_function=OR  inputs=4  en=off  latency=0  precision=Full  arith_type=Unsigned  n_bits=16  bin_pt=0  align_bp=on  overflow=[]  quantization=[]  XmcBlockStatus=1  maskContainerNames=tabcontainer1  block_type=logical  block_config=sysgen:Logical_config
  c_out : hdlBasic/Logical  logical_function=OR  inputs=3  en=off  latency=0  precision=Full  arith_type=Unsigned  n_bits=16  bin_pt=0  align_bp=on  overflow=[]  quantization=[]  XmcBlockStatus=1  maskContainerNames=tabcontainer1  block_type=logical  block_config=sysgen:Logical_config
  ALU_OUT (1 BIT) : Outport
  CARRY_OUT (1 BIT) : Outport  Port=2
  wires:
  A_INPUT (1 BIT)/1 -> Inverter8/1, Logical5/2, Logical/2, Logical2/1, Logical9/2
  Logical1/1 -> c_out/2
  Inverter8/1 -> Logical6/2, Logical4/2
  CARRY_IN (1 BIT)/1 -> Inverter1/1, Logical5/1, Logical4/1, Logical1/1, Logical/1
  B_INPUT (1 BIT)/1 -> Logical5/3, Logical6/3, Logical1/2, Logical2/2, Inverter9/1
  Inverter1/1 -> Logical6/1, Logical9/1
  Logical6/1 -> Sum/3
  Logical9/1 -> Sum/2
  Logical4/1 -> Sum/1
  Logical/1 -> c_out/1
  Logical5/1 -> Sum/4
  Inverter9/1 -> Logical9/3, Logical4/3
  Sum/1 -> ALU_OUT (1 BIT)/1
  Logical2/1 -> c_out/3
  c_out/1 -> CARRY_OUT (1 BIT)/1

== system PROGRAM_COUNTER_02/SUMADOR_64_BITS_1/ALU_SUM_3 ==
  CARRY_IN (1 BIT) : Inport
  A_INPUT (1 BIT) : Inport  Port=2
  B_INPUT (1 BIT) : Inport  Port=3
  Inverter1 : hdlBasic/Inverter  en=off  latency=0  XmcBlockStatus=1  maskContainerNames=group2  block_type=inv  block_config=sysgen:Inverter_config
  Inverter8 : hdlBasic/Inverter  en=off  latency=0  XmcBlockStatus=1  maskContainerNames=group2  block_type=inv  block_config=sysgen:Inverter_config
  Inverter9 : hdlBasic/Inverter  en=off  latency=0  XmcBlockStatus=1  maskContainerNames=group2  block_type=inv  block_config=sysgen:Inverter_config
  Logical : hdlBasic/Logical  logical_function=AND  inputs=2  en=off  latency=0  precision=Full  arith_type=Unsigned  n_bits=16  bin_pt=0  align_bp=on  overflow=[]  quantization=[]  XmcBlockStatus=1  maskContainerNames=tabcontainer1  block_type=logical  block_config=sysgen:Logical_config
  Logical1 : hdlBasic/Logical  logical_function=AND  inputs=2  en=off  latency=0  precision=Full  arith_type=Unsigned  n_bits=16  bin_pt=0  align_bp=on  overflow=[]  quantization=[]  XmcBlockStatus=1  maskContainerNames=tabcontainer1  block_type=logical  block_config=sysgen:Logical_config
  Logical2 : hdlBasic/Logical  logical_function=AND  inputs=2  en=off  latency=0  precision=Full  arith_type=Unsigned  n_bits=16  bin_pt=0  align_bp=on  overflow=[]  quantization=[]  XmcBlockStatus=1  maskContainerNames=tabcontainer1  block_type=logical  block_config=sysgen:Logical_config
  Logical{4..6,9} (4 alike) : hdlBasic/Logical  logical_function=AND  inputs=3  en=off  latency=0  precision=Full  arith_type=Unsigned  n_bits=16  bin_pt=0  align_bp=on  overflow=[]  quantization=[]  XmcBlockStatus=1  maskContainerNames=tabcontainer1  block_type=logical  block_config=sysgen:Logical_config
  Sum : hdlBasic/Logical  logical_function=OR  inputs=4  en=off  latency=0  precision=Full  arith_type=Unsigned  n_bits=16  bin_pt=0  align_bp=on  overflow=[]  quantization=[]  XmcBlockStatus=1  maskContainerNames=tabcontainer1  block_type=logical  block_config=sysgen:Logical_config
  c_out : hdlBasic/Logical  logical_function=OR  inputs=3  en=off  latency=0  precision=Full  arith_type=Unsigned  n_bits=16  bin_pt=0  align_bp=on  overflow=[]  quantization=[]  XmcBlockStatus=1  maskContainerNames=tabcontainer1  block_type=logical  block_config=sysgen:Logical_config
  ALU_OUT (1 BIT) : Outport
  CARRY_OUT (1 BIT) : Outport  Port=2
  wires:
  A_INPUT (1 BIT)/1 -> Inverter8/1, Logical5/2, Logical/2, Logical2/1, Logical9/2
  Logical1/1 -> c_out/2
  Inverter8/1 -> Logical6/2, Logical4/2
  CARRY_IN (1 BIT)/1 -> Inverter1/1, Logical5/1, Logical4/1, Logical1/1, Logical/1
  B_INPUT (1 BIT)/1 -> Logical5/3, Logical6/3, Logical1/2, Logical2/2, Inverter9/1
  Inverter1/1 -> Logical6/1, Logical9/1
  Logical6/1 -> Sum/3
  Logical9/1 -> Sum/2
  Logical4/1 -> Sum/1
  Logical/1 -> c_out/1
  Logical5/1 -> Sum/4
  Inverter9/1 -> Logical9/3, Logical4/3
  Sum/1 -> ALU_OUT (1 BIT)/1
  Logical2/1 -> c_out/3
  c_out/1 -> CARRY_OUT (1 BIT)/1

== system PROGRAM_COUNTER_02/SUMADOR_64_BITS_1/ALU_SUM_30 ==
  CARRY_IN (1 BIT) : Inport
  A_INPUT (1 BIT) : Inport  Port=2
  B_INPUT (1 BIT) : Inport  Port=3
  Inverter1 : hdlBasic/Inverter  en=off  latency=0  XmcBlockStatus=1  maskContainerNames=group2  block_type=inv  block_config=sysgen:Inverter_config
  Inverter8 : hdlBasic/Inverter  en=off  latency=0  XmcBlockStatus=1  maskContainerNames=group2  block_type=inv  block_config=sysgen:Inverter_config
  Inverter9 : hdlBasic/Inverter  en=off  latency=0  XmcBlockStatus=1  maskContainerNames=group2  block_type=inv  block_config=sysgen:Inverter_config
  Logical : hdlBasic/Logical  logical_function=AND  inputs=2  en=off  latency=0  precision=Full  arith_type=Unsigned  n_bits=16  bin_pt=0  align_bp=on  overflow=[]  quantization=[]  XmcBlockStatus=1  maskContainerNames=tabcontainer1  block_type=logical  block_config=sysgen:Logical_config
  Logical1 : hdlBasic/Logical  logical_function=AND  inputs=2  en=off  latency=0  precision=Full  arith_type=Unsigned  n_bits=16  bin_pt=0  align_bp=on  overflow=[]  quantization=[]  XmcBlockStatus=1  maskContainerNames=tabcontainer1  block_type=logical  block_config=sysgen:Logical_config
  Logical2 : hdlBasic/Logical  logical_function=AND  inputs=2  en=off  latency=0  precision=Full  arith_type=Unsigned  n_bits=16  bin_pt=0  align_bp=on  overflow=[]  quantization=[]  XmcBlockStatus=1  maskContainerNames=tabcontainer1  block_type=logical  block_config=sysgen:Logical_config
  Logical{4..6,9} (4 alike) : hdlBasic/Logical  logical_function=AND  inputs=3  en=off  latency=0  precision=Full  arith_type=Unsigned  n_bits=16  bin_pt=0  align_bp=on  overflow=[]  quantization=[]  XmcBlockStatus=1  maskContainerNames=tabcontainer1  block_type=logical  block_config=sysgen:Logical_config
  Sum : hdlBasic/Logical  logical_function=OR  inputs=4  en=off  latency=0  precision=Full  arith_type=Unsigned  n_bits=16  bin_pt=0  align_bp=on  overflow=[]  quantization=[]  XmcBlockStatus=1  maskContainerNames=tabcontainer1  block_type=logical  block_config=sysgen:Logical_config
  c_out : hdlBasic/Logical  logical_function=OR  inputs=3  en=off  latency=0  precision=Full  arith_type=Unsigned  n_bits=16  bin_pt=0  align_bp=on  overflow=[]  quantization=[]  XmcBlockStatus=1  maskContainerNames=tabcontainer1  block_type=logical  block_config=sysgen:Logical_config
  ALU_OUT (1 BIT) : Outport
  CARRY_OUT (1 BIT) : Outport  Port=2
  wires:
  A_INPUT (1 BIT)/1 -> Inverter8/1, Logical5/2, Logical/2, Logical2/1, Logical9/2
  Logical1/1 -> c_out/2
  Inverter8/1 -> Logical6/2, Logical4/2
  CARRY_IN (1 BIT)/1 -> Inverter1/1, Logical5/1, Logical4/1, Logical1/1, Logical/1
  B_INPUT (1 BIT)/1 -> Logical5/3, Logical6/3, Logical1/2, Logical2/2, Inverter9/1
  Inverter1/1 -> Logical6/1, Logical9/1
  Logical6/1 -> Sum/3
  Logical9/1 -> Sum/2
  Logical4/1 -> Sum/1
  Logical/1 -> c_out/1
  Logical5/1 -> Sum/4
  Inverter9/1 -> Logical9/3, Logical4/3
  Sum/1 -> ALU_OUT (1 BIT)/1
  Logical2/1 -> c_out/3
  c_out/1 -> CARRY_OUT (1 BIT)/1

== system PROGRAM_COUNTER_02/SUMADOR_64_BITS_1/ALU_SUM_31 ==
  CARRY_IN (1 BIT) : Inport
  A_INPUT (1 BIT) : Inport  Port=2
  B_INPUT (1 BIT) : Inport  Port=3
  Inverter1 : hdlBasic/Inverter  en=off  latency=0  XmcBlockStatus=1  maskContainerNames=group2  block_type=inv  block_config=sysgen:Inverter_config
  Inverter8 : hdlBasic/Inverter  en=off  latency=0  XmcBlockStatus=1  maskContainerNames=group2  block_type=inv  block_config=sysgen:Inverter_config
  Inverter9 : hdlBasic/Inverter  en=off  latency=0  XmcBlockStatus=1  maskContainerNames=group2  block_type=inv  block_config=sysgen:Inverter_config
  Logical : hdlBasic/Logical  logical_function=AND  inputs=2  en=off  latency=0  precision=Full  arith_type=Unsigned  n_bits=16  bin_pt=0  align_bp=on  overflow=[]  quantization=[]  XmcBlockStatus=1  maskContainerNames=tabcontainer1  block_type=logical  block_config=sysgen:Logical_config
  Logical1 : hdlBasic/Logical  logical_function=AND  inputs=2  en=off  latency=0  precision=Full  arith_type=Unsigned  n_bits=16  bin_pt=0  align_bp=on  overflow=[]  quantization=[]  XmcBlockStatus=1  maskContainerNames=tabcontainer1  block_type=logical  block_config=sysgen:Logical_config
  Logical2 : hdlBasic/Logical  logical_function=AND  inputs=2  en=off  latency=0  precision=Full  arith_type=Unsigned  n_bits=16  bin_pt=0  align_bp=on  overflow=[]  quantization=[]  XmcBlockStatus=1  maskContainerNames=tabcontainer1  block_type=logical  block_config=sysgen:Logical_config
  Logical{4..6,9} (4 alike) : hdlBasic/Logical  logical_function=AND  inputs=3  en=off  latency=0  precision=Full  arith_type=Unsigned  n_bits=16  bin_pt=0  align_bp=on  overflow=[]  quantization=[]  XmcBlockStatus=1  maskContainerNames=tabcontainer1  block_type=logical  block_config=sysgen:Logical_config
  Sum : hdlBasic/Logical  logical_function=OR  inputs=4  en=off  latency=0  precision=Full  arith_type=Unsigned  n_bits=16  bin_pt=0  align_bp=on  overflow=[]  quantization=[]  XmcBlockStatus=1  maskContainerNames=tabcontainer1  block_type=logical  block_config=sysgen:Logical_config
  c_out : hdlBasic/Logical  logical_function=OR  inputs=3  en=off  latency=0  precision=Full  arith_type=Unsigned  n_bits=16  bin_pt=0  align_bp=on  overflow=[]  quantization=[]  XmcBlockStatus=1  maskContainerNames=tabcontainer1  block_type=logical  block_config=sysgen:Logical_config
  ALU_OUT (1 BIT) : Outport
  CARRY_OUT (1 BIT) : Outport  Port=2
  wires:
  A_INPUT (1 BIT)/1 -> Inverter8/1, Logical5/2, Logical/2, Logical2/1, Logical9/2
  Logical1/1 -> c_out/2
  Inverter8/1 -> Logical6/2, Logical4/2
  CARRY_IN (1 BIT)/1 -> Inverter1/1, Logical5/1, Logical4/1, Logical1/1, Logical/1
  B_INPUT (1 BIT)/1 -> Logical5/3, Logical6/3, Logical1/2, Logical2/2, Inverter9/1
  Inverter1/1 -> Logical6/1, Logical9/1
  Logical6/1 -> Sum/3
  Logical9/1 -> Sum/2
  Logical4/1 -> Sum/1
  Logical/1 -> c_out/1
  Logical5/1 -> Sum/4
  Inverter9/1 -> Logical9/3, Logical4/3
  Sum/1 -> ALU_OUT (1 BIT)/1
  Logical2/1 -> c_out/3
  c_out/1 -> CARRY_OUT (1 BIT)/1
